simulink model "Punto_7"  (R2022a)
settings: Solver=VariableStepAuto  StartTime=0.0  StopTime=10.0  RelTol=1e-3
undefined symbols (not defined in the file): A, B, t0
libraries: simulink x3
settings Model: Creator=garzo  LastModifiedBy=garzo

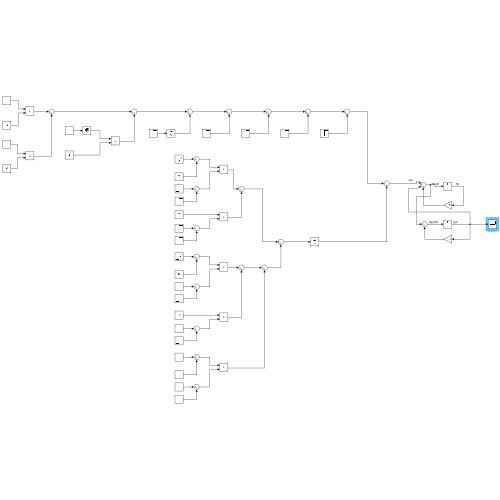
[thumbnail: Simulink's stored preview of the top-level diagram]
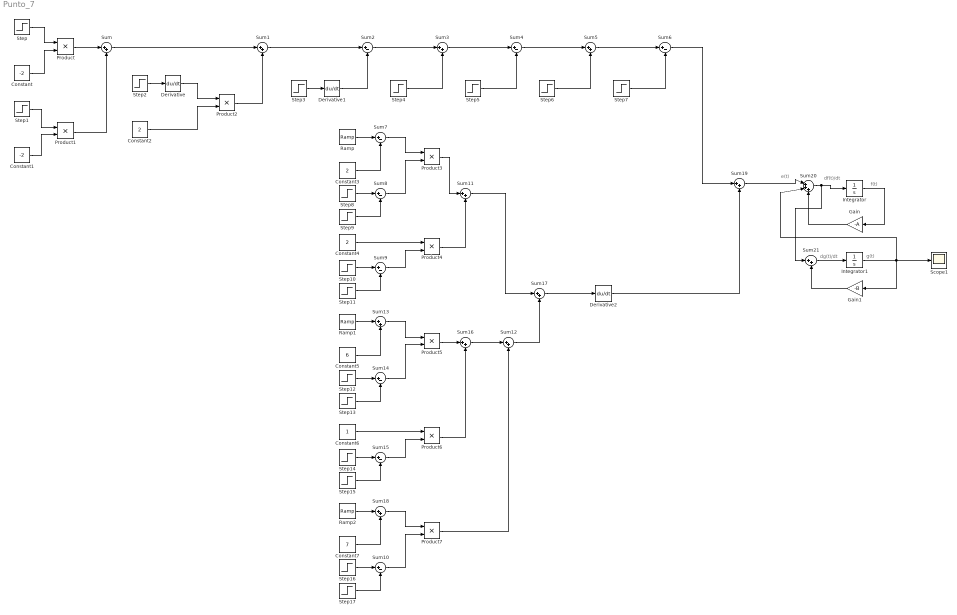
== system Punto_7 ==
  note: e(t)
  note: g(t)
  note: f(t)
  note: dg(t)/dt
  note: df(t)/dt
  Constant : Constant  Value=-2
  Constant1 : Constant  Value=-2
  Constant2 : Constant  Value=2
  Constant3 : Constant  Value=2
  Constant4 : Constant  Value=2
  Constant5 : Constant  Value=6
  Constant6 : Constant
  Constant7 : Constant  Value=7
  Derivative : Derivative
  Derivative1 : Derivative
  Derivative2 : Derivative
  Gain : Gain  Gain=-A
  Gain1 : Gain  Gain=-B
  Integrator : Integrator
  Integrator1 : Integrator
  Product{,1..7} (8 alike) : Product
  Ramp : simulink/Sources/Ramp  slope=2  start=t0  InitialOutput=0
  Ramp1 : simulink/Sources/Ramp  slope=-1  start=t0  InitialOutput=0
  Ramp2 : simulink/Sources/Ramp  slope=-1  start=t0  InitialOutput=0
  Scope1 : Scope
  Step : Step  Time=0  SampleTime=0
  Step1 : Step  Time=2  SampleTime=0
  Step10 : Step  Time=t0+2  SampleTime=0
  Step11 : Step  Time=t0+3  SampleTime=0
  Step12 : Step  Time=t0+3  SampleTime=0
  Step13 : Step  Time=t0+5  SampleTime=0
  Step14 : Step  Time=t0+5  SampleTime=0
  Step15 : Step  Time=t0+6  SampleTime=0
  Step16 : Step  Time=t0+6  SampleTime=0
  Step17 : Step  Time=t0+8  SampleTime=0
  Step2 : Step  Time=0  SampleTime=0
  Step3 : Step  Time=8  SampleTime=0
  Step4 : Step  Time=3  SampleTime=0
  Step5 : Step  Time=5  SampleTime=0
  Step6 : Step  Time=6  SampleTime=0
  Step7 : Step  Time=8  SampleTime=0
  Step8 : Step  Time=t0  SampleTime=0
  Step9 : Step  Time=t0+2  SampleTime=0
  Sum{,1,3,5,11..13,16..19,21} (12 alike) : Sum  Inputs=|++
  Sum{2,4,6..10,14..15} (9 alike) : Sum  Inputs=|+-
  Sum20 : Sum  Inputs=|+++
  wires:
  Step17/1 -> Sum10/2
  Step12/1 -> Sum14/1
  Sum17/1 -> Derivative2/1
  Step16/1 -> Sum10/1
  Step3/1 -> Derivative1/1
  Sum6/1 -> Sum19/1
  Sum2/1 -> Sum3/1
  Step11/1 -> Sum9/2
  Derivative2/1 -> Sum19/2
  Sum16/1 -> Sum12/1
  Constant5/1 -> Sum13/2
  Step13/1 -> Sum14/2
  Product1/1 -> Sum/2
  Sum14/1 -> Product5/2
  Sum13/1 -> Product5/1
  Sum10/1 -> Product7/2
  Constant4/1 -> Product4/1
  Product3/1 -> Sum11/1
  Step10/1 -> Sum9/1
  Sum12/1 -> Sum17/2
  Constant3/1 -> Sum7/2
  Sum9/1 -> Product4/2
  Product5/1 -> Sum16/1
  Sum7/1 -> Product3/1
  Ramp/1 -> Sum7/1
  Step6/1 -> Sum5/2
  Sum5/1 -> Sum6/1
  Step1/1 -> Product1/1
  Sum8/1 -> Product3/2
  Step7/1 -> Sum6/2
  Sum11/1 -> Sum17/1
  Derivative1/1 -> Sum2/2
  Derivative/1 -> Product2/1
  Step9/1 -> Sum8/2
  Sum15/1 -> Product6/2
  Product7/1 -> Sum12/2
  Ramp2/1 -> Sum18/1
  Step15/1 -> Sum15/2
  Constant6/1 -> Product6/1
  Step5/1 -> Sum4/2
  Ramp1/1 -> Sum13/1
  Product4/1 -> Sum11/2
  Sum4/1 -> Sum5/1
  Step8/1 -> Sum8/1
  Sum3/1 -> Sum4/1
  Sum18/1 -> Product7/1
  Step/1 -> Product/1
  Constant/1 -> Product/2
  Constant2/1 -> Product2/2
  Product6/1 -> Sum16/2
  Constant7/1 -> Sum18/2
  Step2/1 -> Derivative/1
  Product2/1 -> Sum1/2
  Sum1/1 -> Sum2/1
  Product/1 -> Sum/1
  Step14/1 -> Sum15/1
  Constant1/1 -> Product1/2
  Step4/1 -> Sum3/2
  Sum/1 -> Sum1/1
  Gain1/1 -> Sum21/2
  Sum21/1 -> Integrator1/1
  Integrator/1 -> Gain/1
  Integrator1/1 -> Sum20/2, Scope1/1, Gain1/1
  Sum20/1 -> Sum21/1, Integrator/1
  Gain/1 -> Sum20/3
  Sum19/1 -> Sum20/1
